simulink model "OL_HiLData"  (R2015b)
settings: Solver=FixedStepDiscrete  StartTime=0.0  StopTime=660  FixedStep=step_size  RelTol=1e-3
values from neighbouring files (symbols this model uses):
  step_size = 0.1    [loadCalib.m]
undefined symbols (not defined in the file or in its folder): canChannel, pack_current_eng, pack_current_raw, pack_voltage_eng, pack_voltage_raw, vehicle_voltage_eng, vehicle_voltage_raw
libraries: canmsglib x34, canlib x27, realtime_pacer_lib x1
(part 1 of 2)
settings Model: SimulationMode=accelerator  Creator=nctzv8  LastModifiedBy=nctzv8

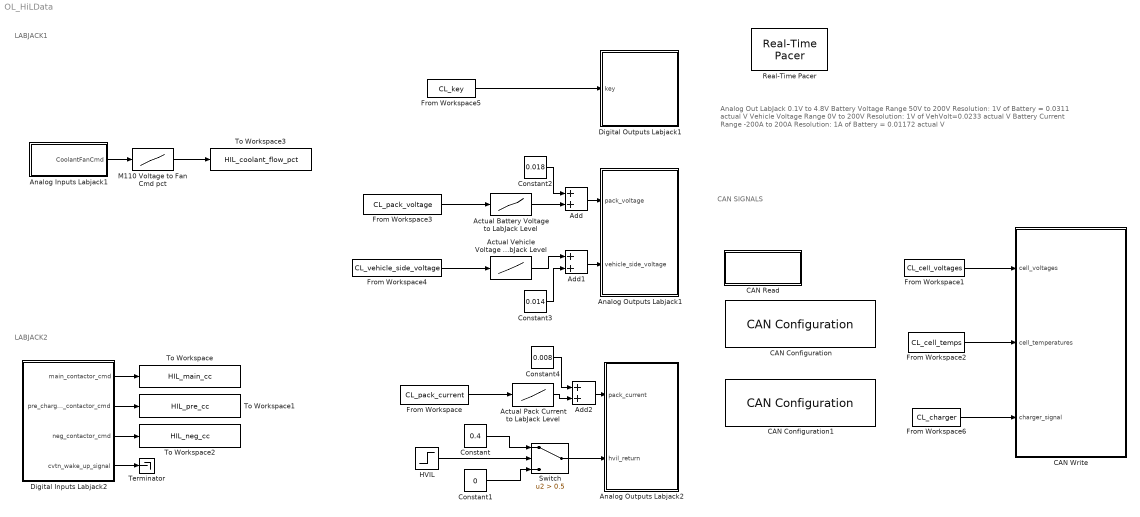
== system OL_HiLData ==
  note: CAN SIGNALS
  note: LABJACK2
  note: LABJACK1
  note: Analog Out LabJack 0.1V to 4.8V
      | Battery Voltage Range 50V to 200V Resolution: 1V of Battery = 0.0311 actual V
      | Vehicle Voltage Range 0V to 200V Resolution: 1V of VehVolt=0.0233 actual V
      | Battery Current Range -200A to 200A Resolution: 1A of Battery = 0.01172 actual V
  Actual Battery Voltage to LabJack Level : Lookup_n-D  NumberOfTableDimensions=1  BreakpointsForDimension1=pack_voltage_eng  Table=pack_voltage_raw  InternalRulePriority=Speed  RndMeth=Simplest  InputSameDT=on
  Actual Pack Current to LabJack Level : Lookup_n-D  NumberOfTableDimensions=1  BreakpointsForDimension1=pack_current_eng  Table=pack_current_raw  InternalRulePriority=Speed  RndMeth=Simplest  InputSameDT=on
  Actual Vehicle Voltage to LabJack Level : Lookup_n-D  NumberOfTableDimensions=1  BreakpointsForDimension1=vehicle_voltage_eng  Table=vehicle_voltage_raw  InternalRulePriority=Speed  RndMeth=Simplest  InputSameDT=on
  Add : Sum
  Add1 : Sum
  Add2 : Sum
  Analog Inputs Labjack1 : Subsystem
  Analog Outputs Labjack1 : Subsystem
  Analog Outputs Labjack2 : Subsystem
  CAN Configuration : canlib/CAN Configuration  BlockHandle=54.0011  DeviceMenu=Kvaser Virtual 1 (Channel 1)  Device=Kvaser USBcan Light 2 (Channel 1)  ObjConstructor=canChannel('Kvaser', 'USBcan Light 2', 1)  BusSpeed=500000  EnableBitParameters=off  SJW=1  TSEG1=4  TSEG2=3  NSamples=1  AckMode=Normal
  CAN Configuration1 : canlib/CAN Configuration  BlockHandle=55.0007  DeviceMenu=Kvaser Virtual 1 (Channel 1)  Device=Kvaser USBcan Light 2 (Channel 2)  ObjConstructor=canChannel('Kvaser', 'USBcan Light 2', 2)  BusSpeed=500000  EnableBitParameters=off  SJW=1  TSEG1=4  TSEG2=3  NSamples=1  AckMode=Normal
  CAN Read : Subsystem
  CAN Write : Subsystem
  Constant : Constant  Value=0.4  SampleTime=step_size
  Constant1 : Constant  Value=0  SampleTime=step_size
  Constant2 : Constant  Value=0.018  SampleTime=step_size
  Constant3 : Constant  Value=0.014  SampleTime=step_size
  Constant4 : Constant  Value=0.008  SampleTime=step_size
  Digital Inputs Labjack2 : Subsystem
  Digital Outputs Labjack1 : Subsystem
  From Workspace : FromWorkspace  VariableName=CL_pack_current  SampleTime=step_size
  From Workspace1 : FromWorkspace  VariableName=CL_cell_voltages  SampleTime=step_size
  From Workspace2 : FromWorkspace  VariableName=CL_cell_temps  SampleTime=step_size
  From Workspace3 : FromWorkspace  VariableName=CL_pack_voltage  SampleTime=step_size
  From Workspace4 : FromWorkspace  VariableName=CL_vehicle_side_voltage  SampleTime=step_size
  From Workspace5 : FromWorkspace  VariableName=CL_key  SampleTime=step_size
  From Workspace6 : FromWorkspace  VariableName=CL_charger  SampleTime=step_size
  HVIL : Step  Time=0  Before=1  SampleTime=step_size
  M110 Voltage to Fan Cmd pct : Lookup_n-D  NumberOfTableDimensions=1  BreakpointsForDimension1=[0 5]  Table=[0 100]  InternalRulePriority=Speed  RndMeth=Simplest  InputSameDT=on
  Real-Time Pacer : realtime_pacer_lib/Real-Time Pacer  simTimePerRealTime=1
  Switch : Switch  Criteria=u2 > Threshold  Threshold=0.5
  Terminator : Terminator
  To Workspace : ToWorkspace  VariableName=HIL_main_cc  SaveFormat=Timeseries  SampleTime=-1
  To Workspace1 : ToWorkspace  VariableName=HIL_pre_cc  SaveFormat=Timeseries  SampleTime=-1
  To Workspace2 : ToWorkspace  VariableName=HIL_neg_cc  SaveFormat=Timeseries  SampleTime=-1
  To Workspace3 : ToWorkspace  VariableName=HIL_coolant_flow_pct  SaveFormat=Timeseries  SampleTime=-1
  wires:
  From Workspace3/1 -> Actual Battery Voltage to LabJack Level/1
  From Workspace4/1 -> Actual Vehicle Voltage to LabJack Level/1
  From Workspace/1 -> Actual Pack Current to LabJack Level/1
  From Workspace5/1 -> Digital Outputs Labjack1/1(key)
  From Workspace1/1 -> CAN Write/1(cell_voltages)
  From Workspace2/1 -> CAN Write/2(cell_temperatures)
  HVIL/1 -> Switch/2
  Constant/1 -> Switch/1
  Constant1/1 -> Switch/3
  Switch/1 -> Analog Outputs Labjack2/2(hvil_return)
  Add/1 -> Analog Outputs Labjack1/1(pack_voltage)
  Actual Battery Voltage to LabJack Level/1 -> Add/2
  Constant2/1 -> Add/1
  Add1/1 -> Analog Outputs Labjack1/2(vehicle_side_voltage)
  Actual Vehicle Voltage to LabJack Level/1 -> Add1/1
  Constant3/1 -> Add1/2
  Add2/1 -> Analog Outputs Labjack2/1(pack_current)
  Actual Pack Current to LabJack Level/1 -> Add2/2
  Constant4/1 -> Add2/1
  Digital Inputs Labjack2/1(main_contactor_cmd) -> To Workspace/1
  Digital Inputs Labjack2/2(pre_charge_contactor_cmd) -> To Workspace1/1
  Digital Inputs Labjack2/3(neg_contactor_cmd) -> To Workspace2/1
  Digital Inputs Labjack2/4(cvtn_wake_up_signal) -> Terminator/1
  From Workspace6/1 -> CAN Write/3(charger_signal)
  Analog Inputs Labjack1/1(CoolantFanCmd) -> M110 Voltage to Fan Cmd pct/1
  M110 Voltage to Fan Cmd pct/1 -> To Workspace3/1

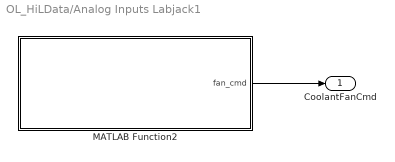
== system OL_HiLData/Analog Inputs Labjack1 ==
  MATLAB Function2 : MATLAB Function  TreatAsAtomicUnit=on
  CoolantFanCmd : Outport
  wires:
  MATLAB Function2/1(fan_cmd) -> CoolantFanCmd/1

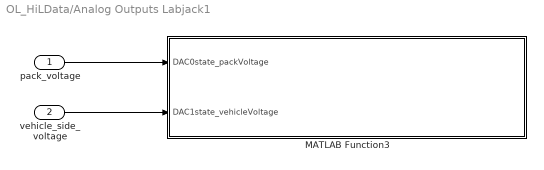
== system OL_HiLData/Analog Outputs Labjack1 ==
  pack_voltage : Inport
  vehicle_side_voltage : Inport  Port=2
  MATLAB Function3 : MATLAB Function  TreatAsAtomicUnit=on
  wires:
  pack_voltage/1 -> MATLAB Function3/1(DAC0state_packVoltage)
  vehicle_side_voltage/1 -> MATLAB Function3/2(DAC1state_vehicleVoltage)

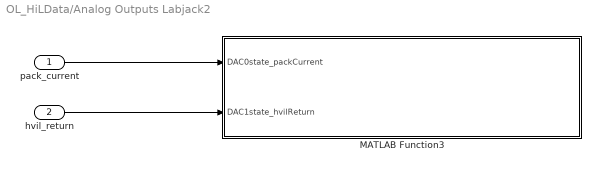
== system OL_HiLData/Analog Outputs Labjack2 ==
  pack_current : Inport
  hvil_return : Inport  Port=2
  MATLAB Function3 : MATLAB Function  TreatAsAtomicUnit=on
  wires:
  pack_current/1 -> MATLAB Function3/1(DAC0state_packCurrent)
  hvil_return/1 -> MATLAB Function3/2(DAC1state_hvilReturn)

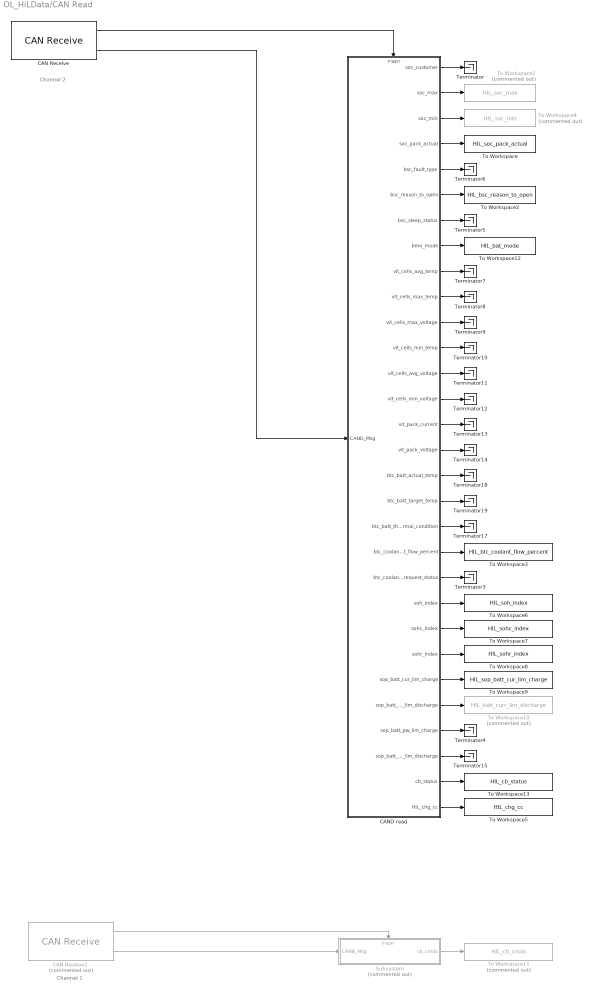
== system OL_HiLData/CAN Read ==
  note: Channel 1
  note: Channel 2
  CAN Receive : canlib/CAN Receive  BlockHandle=57.0007  DeviceMenu=Kvaser Virtual 1 (Channel 1)  Device=Kvaser USBcan Light 2 (Channel 2)  ObjConstructor=canChannel('Kvaser', 'USBcan Light 2', 2)  EnableStandardIDsFilter=off  StandardIDs=0  EnableExtendedIDsFilter=off  ExtendedIDs=0  SampleTime=step_size  MsgsPerTimestep=all  StdIDsCombo=Allow all  ExtIDsCombo=Allow all  InternalFilterUpdateStatus=on
  CAN Receive1 : canlib/CAN Receive  Commented=on  BlockHandle=58.0006  DeviceMenu=Kvaser Virtual 1 (Channel 1)  Device=Kvaser USBcan Light 2 (Channel 1)  ObjConstructor=canChannel('Kvaser', 'USBcan Light 2', 1)  EnableStandardIDsFilter=off  StandardIDs=0  EnableExtendedIDsFilter=off  ExtendedIDs=0  SampleTime=step_size  MsgsPerTimestep=all  StdIDsCombo=Allow all  ExtIDsCombo=Allow all  InternalFilterUpdateStatus=on
  CAND read : Subsystem
  Subsystem : Subsystem  Commented=on
  Terminator{,3..15,17..19} (17 alike) : Terminator
  To Workspace : ToWorkspace  VariableName=HIL_soc_pack_actual  SaveFormat=Timeseries  SampleTime=-1
  To Workspace1 : ToWorkspace  Commented=on  VariableName=HIL_soc_max  SaveFormat=Timeseries  SampleTime=-1
  To Workspace10 : ToWorkspace  Commented=on  VariableName=HIL_batt_curr_lim_discharge  SaveFormat=Timeseries  SampleTime=-1
  To Workspace11 : ToWorkspace  Commented=on  VariableName=HIL_cb_cmds  SaveFormat=Timeseries  SampleTime=-1
  To Workspace12 : ToWorkspace  VariableName=HIL_bat_mode  SaveFormat=Timeseries  SampleTime=-1
  To Workspace13 : ToWorkspace  VariableName=HIL_cb_status  SaveFormat=Timeseries  SampleTime=-1
  To Workspace2 : ToWorkspace  VariableName=HIL_bsc_reason_to_open  SaveFormat=Timeseries  SampleTime=-1
  To Workspace3 : ToWorkspace  VariableName=HIL_btc_coolant_flow_percent  SaveFormat=Timeseries  SampleTime=-1
  To Workspace4 : ToWorkspace  Commented=on  VariableName=HIL_soc_min  SaveFormat=Timeseries  SampleTime=-1
  To Workspace5 : ToWorkspace  VariableName=HIL_chg_cc  SaveFormat=Timeseries  SampleTime=-1
  To Workspace6 : ToWorkspace  VariableName=HIL_soh_index  SaveFormat=Timeseries  SampleTime=-1
  To Workspace7 : ToWorkspace  VariableName=HIL_sohc_index  SaveFormat=Timeseries  SampleTime=-1
  To Workspace8 : ToWorkspace  VariableName=HIL_sohr_index  SaveFormat=Timeseries  SampleTime=-1
  To Workspace9 : ToWorkspace  VariableName=HIL_sop_batt_cur_lim_charge  SaveFormat=Timeseries  SampleTime=-1
  wires:
  CAN Receive/2 -> CAND read/1(CAND_Msg)
  CAND read/1(soc_customer) -> Terminator/1
  CAND read/2(soc_max) -> To Workspace1/1
  CAND read/3(soc_min) -> To Workspace4/1
  CAND read/4(soc_pack_actual) -> To Workspace/1
  CAND read/5(bsc_fault_type) -> Terminator6/1
  CAND read/6(bsc_reason_to_open) -> To Workspace2/1
  CAND read/7(bsc_sleep_status) -> Terminator5/1
  CAND read/8(bmo_mode) -> To Workspace12/1
  CAND read/9(vit_cells_avg_temp) -> Terminator7/1
  CAND read/10(vit_cells_max_temp) -> Terminator8/1
  CAND read/11(vit_cells_max_voltage) -> Terminator9/1
  CAND read/12(vit_cells_min_temp) -> Terminator10/1
  CAND read/13(vit_cells_avg_voltage) -> Terminator11/1
  CAND read/14(vit_cells_min_voltage) -> Terminator12/1
  CAND read/15(vit_pack_current) -> Terminator13/1
  CAND read/16(vit_pack_voltage) -> Terminator14/1
  CAND read/17(btc_batt_actual_temp) -> Terminator18/1
  CAND read/18(btc_batt_target_temp) -> Terminator19/1
  CAND read/19(btc_batt_thermal_condition) -> Terminator17/1
  CAND read/20(btc_coolant_flow_percent) -> To Workspace3/1
  CAND read/21(btc_coolant_request_status) -> Terminator3/1
  CAND read/22(soh_index) -> To Workspace6/1
  CAND read/23(sohc_index) -> To Workspace7/1
  CAND read/24(sohr_index) -> To Workspace8/1
  CAND read/25(sop_batt_cur_lim_charge) -> To Workspace9/1
  CAND read/26(sop_batt_curr_lim_discharge) -> To Workspace10/1
  CAND read/27(sop_batt_pw_lim_charge) -> Terminator4/1
  CAND read/28(sop_batt_pw_lim_discharge) -> Terminator15/1
  CAND read/29(cb_status) -> To Workspace13/1
  CAN Receive1/1 -> Subsystem/Trigger
  CAN Receive1/2 -> Subsystem/1(CANB_Msg)
  Subsystem/1(cb_cmds) -> To Workspace11/1
  CAND read/30(HIL_chg_cc) -> To Workspace5/1
  CAN Receive/1 -> CAND read/Trigger

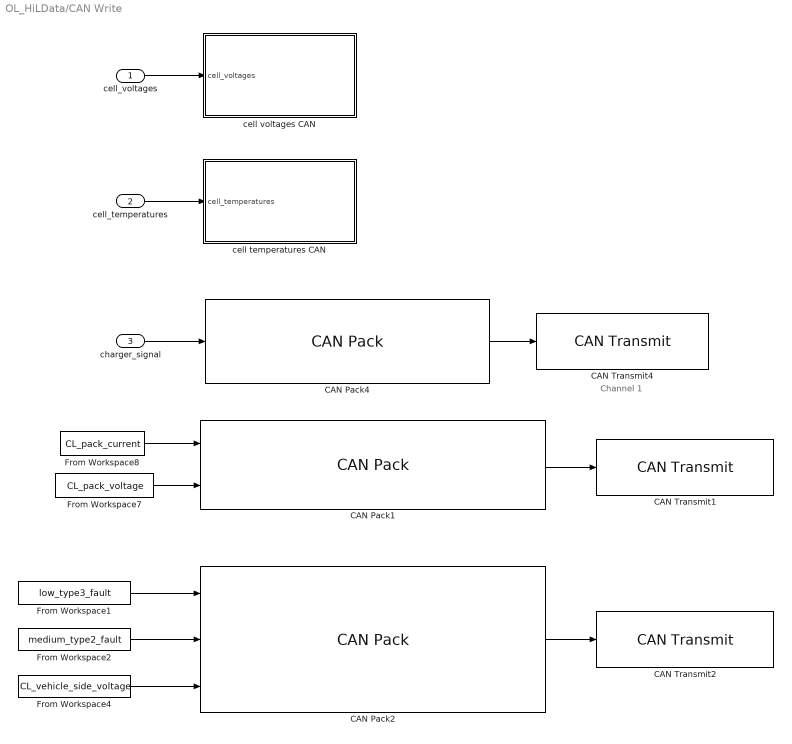
== system OL_HiLData/CAN Write ==
  note: Channel 1
  cell_voltages : Inport
  cell_temperatures : Inport  Port=2
  charger_signal : Inport  Port=3
  CAN Pack1 : canmsglib/CAN Pack  CANdbFile=C:\Sagar\Projects\BMS\P006n\08_Work_in_progress\WP3_2_BMS_Stage_1\OpenLoopDataSend\BMSdb.dbc  MsgList=pack_data  MsgName=pack_data  MsgIDType=Standard (11-bit identifier)  MsgIdentifier=36  MsgLength=8  SignalInfo=pack_current$16$24$2$1$1$0$1.000000e-03$0$-200$200$#pack_voltage$40$24$2$2$1$0$1.000000e-03$0$0$200$#  NSignals=2  StartBits=str2num('[int32(16);int32(40)]')  SignalSizes=str2num('[int32(24);int32(24)]')  ByteOrders=str2num('[int32(2);int32(2)]')  DataTypes=str2num('[int32(1);int32(2)]')  MultiplexTypes=str2num('[int32(1);int32(1)]')  MultiplexValues=str2num('[double(0);double(0)]')  Factors=str2num('[double(1.000000e-03);double(1.000000e-03)]')  Offsets=str2num('[double(0);double(0)]')  Minimums=str2num('[double(-200);double(0)]')  Maximums=str2num('[double(200);double(200)]')  Remote=off
      settings: DataFormat=CANdb specified signals
  CAN Pack2 : canmsglib/CAN Pack  CANdbFile=C:\Sagar\Projects\BMS\P006n\08_Work_in_progress\WP3_2_BMS_Stage_1\OpenLoopDataSend\BMSdb.dbc  MsgList=pack_data_2  MsgName=pack_data_2  MsgIDType=Standard (11-bit identifier)  MsgIdentifier=37  MsgLength=8  SignalInfo=low_fault$30$1$2$2$1$0$1$0$0$1$#medium_fault$31$1$2$2$1$0$1$0$0$1$#vehicle_side_voltage$16$24$2$2$1$0$1$0$0$200$#  NSignals=3  StartBits=str2num('[int32(30);int32(31);int32(16)]')  SignalSizes=str2num('[int32(1);int32(1);int32(24)]')  ByteOrders=str2num('[int32(2);int32(2);int32(2)]')  DataTypes=str2num('[int32(2);int32(2);int32(2)]')  MultiplexTypes=str2num('[int32(1);int32(1);int32(1)]')  MultiplexValues=str2num('[double(0);double(0);double(0)]')  Factors=str2num('[double(1);double(1);double(1)]')  Offsets=str2num('[double(0);double(0);double(0)]')  Minimums=str2num('[double(0);double(0);double(0)]')  Maximums=str2num('[double(1);double(1);double(200)]')  Remote=off
      settings: DataFormat=CANdb specified signals
  CAN Pack4 : canmsglib/CAN Pack  CANdbFile=C:\Sagar\Projects\BMS\P006n\08_Work_in_progress\WP3_2_BMS_Stage_1\OpenLoopDataSend\BMSdb.dbc  MsgList=socket_charging  MsgName=socket_charging  MsgIDType=Standard (11-bit identifier)  MsgIdentifier=35  MsgLength=8  SignalInfo=charger_signal$7$1$2$2$1$0$1$0$0$1$#  NSignals=1  StartBits=str2num('[int32(7)]')  SignalSizes=str2num('[int32(1)]')  ByteOrders=str2num('[int32(2)]')  DataTypes=str2num('[int32(2)]')  MultiplexTypes=str2num('[int32(1)]')  MultiplexValues=str2num('[double(0)]')  Factors=str2num('[double(1)]')  Offsets=str2num('[double(0)]')  Minimums=str2num('[double(0)]')  Maximums=str2num('[double(1)]')  Remote=off
      settings: DataFormat=CANdb specified signals
  CAN Transmit1 : canlib/CAN Transmit  BlockHandle=300.0009  DeviceMenu=Kvaser Virtual 1 (Channel 1)  Device=Kvaser USBcan Light 2 (Channel 1)  ObjConstructor=canChannel('Kvaser', 'USBcan Light 2', 1)  EnablePeriodicTransmit=off  MessagePeriod=1.000
  CAN Transmit2 : canlib/CAN Transmit  BlockHandle=301.0009  DeviceMenu=Kvaser Virtual 1 (Channel 1)  Device=Kvaser USBcan Light 2 (Channel 1)  ObjConstructor=canChannel('Kvaser', 'USBcan Light 2', 1)  EnablePeriodicTransmit=off  MessagePeriod=1.000
  CAN Transmit4 : canlib/CAN Transmit  BlockHandle=302.0009  DeviceMenu=Kvaser Virtual 1 (Channel 1)  Device=Kvaser USBcan Light 2 (Channel 1)  ObjConstructor=canChannel('Kvaser', 'USBcan Light 2', 1)  EnablePeriodicTransmit=off  MessagePeriod=1.000
  From Workspace1 : FromWorkspace  VariableName=low_type3_fault  SampleTime=step_size
  From Workspace2 : FromWorkspace  VariableName=medium_type2_fault  SampleTime=step_size
  From Workspace4 : FromWorkspace  VariableName=CL_vehicle_side_voltage  SampleTime=step_size
  From Workspace7 : FromWorkspace  VariableName=CL_pack_voltage  SampleTime=step_size
  From Workspace8 : FromWorkspace  VariableName=CL_pack_current  SampleTime=step_size
  cell temperatures CAN : Subsystem
  cell voltages CAN : Subsystem
  wires:
  cell_voltages/1 -> cell voltages CAN/1(cell_voltages)
  cell_temperatures/1 -> cell temperatures CAN/1(cell_temperatures)
  CAN Pack4/1 -> CAN Transmit4/1
  charger_signal/1 -> CAN Pack4/1
  CAN Pack1/1 -> CAN Transmit1/1
  From Workspace8/1 -> CAN Pack1/1
  From Workspace7/1 -> CAN Pack1/2
  CAN Pack2/1 -> CAN Transmit2/1
  From Workspace4/1 -> CAN Pack2/3
  From Workspace1/1 -> CAN Pack2/1
  From Workspace2/1 -> CAN Pack2/2

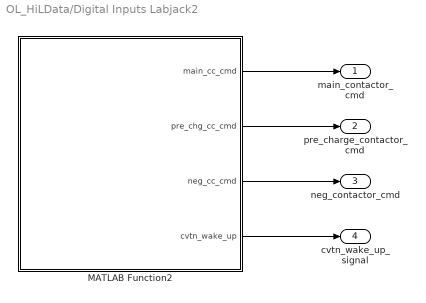
== system OL_HiLData/Digital Inputs Labjack2 ==
  MATLAB Function2 : MATLAB Function  TreatAsAtomicUnit=on
  main_contactor_cmd : Outport
  pre_charge_contactor_cmd : Outport  Port=2
  neg_contactor_cmd : Outport  Port=3
  cvtn_wake_up_signal : Outport  Port=4
  wires:
  MATLAB Function2/1(main_cc_cmd) -> main_contactor_cmd/1
  MATLAB Function2/2(pre_chg_cc_cmd) -> pre_charge_contactor_cmd/1
  MATLAB Function2/3(neg_cc_cmd) -> neg_contactor_cmd/1
  MATLAB Function2/4(cvtn_wake_up) -> cvtn_wake_up_signal/1

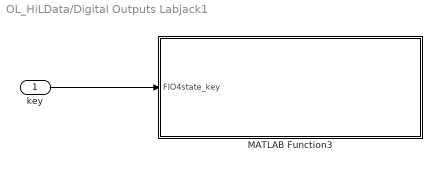
== system OL_HiLData/Digital Outputs Labjack1 ==
  key : Inport
  MATLAB Function3 : MATLAB Function  TreatAsAtomicUnit=on
  wires:
  key/1 -> MATLAB Function3/1(FIO4state_key)

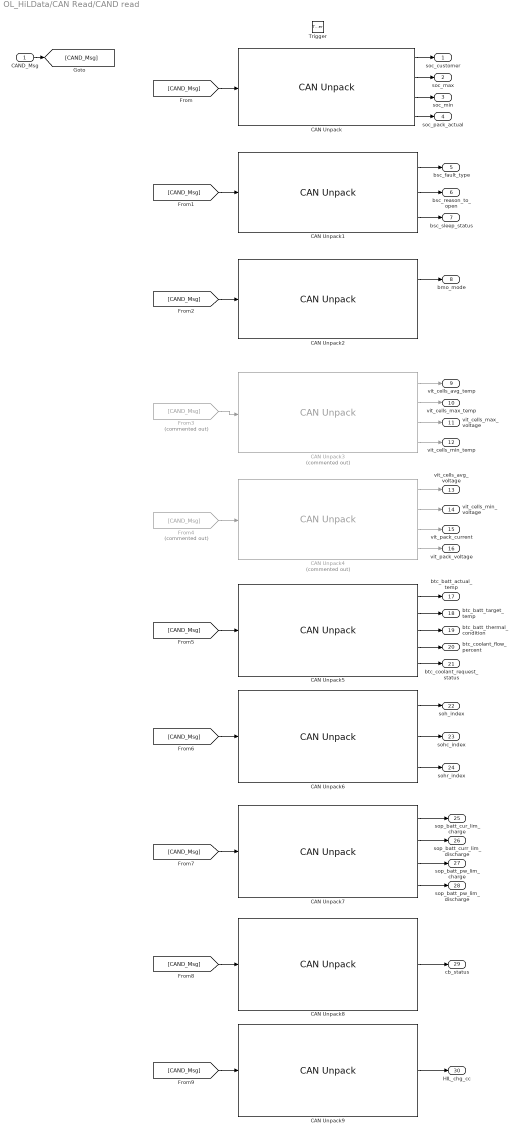
== system OL_HiLData/CAN Read/CAND read ==
  CAND_Msg : Inport
  Trigger : TriggerPort  TriggerType=function-call  PortDimensions=1
  CAN Unpack : canmsglib/CAN Unpack  CANdbFile=C:\Sagar\Projects\BMS\P006n\08_Work_in_progress\WP3_2_BMS_Stage_1\OpenLoopDataSend\VEHdb.dbc  MsgList=soc_info  MsgName=soc_info  MsgIDType=Standard (11-bit identifier)  MsgIdentifier=2  MsgLength=8  SignalInfo=soc_customer$8$16$2$2$1$0$1.000000e-02$0$0$100$#soc_max$56$16$2$2$1$0$1.000000e-02$0$0$100$#soc_min$40$16$2$2$1$0$1.000000e-02$0$0$100$#soc_pack_actual$24$16$2$2$1$0$1.000000e-02$0$0$100$#  NSignals=4  IDPort=off  TimestampPort=off  ErrorPort=off  RemotePort=off  LengthPort=off  StatusPort=off  StartBits=str2num('[int32(8);int32(56);int32(40);int32(24)]')  SignalSizes=str2num('[int32(16);int32(16);int32(16);int32(16)]')  ByteOrders=str2num('[int32(2);int32(2);int32(2);int32(2)]')  DataTypes=str2num('[int32(2);int32(2);int32(2);int32(2)]')  MultiplexTypes=str2num('[int32(1);int32(1);int32(1);int32(1)]')  MultiplexValues=str2num('[double(0);double(0);double(0);double(0)]')  Factors=str2num('[double(1.000000e-02);double(1.000000e-02);double(1.000000e-02);double(1.000000e-02)]')  Offsets=str2num('[double(0);double(0);double(0);double(0)]')  Minimums=str2num('[double(0);double(0);double(0);double(0)]')  Maximums=str2num('[double(100);double(100);double(100);double(100)]')
      settings: DataFormat=CANdb specified signals
  CAN Unpack1 : canmsglib/CAN Unpack  CANdbFile=C:\Sagar\Projects\BMS\P006n\08_Work_in_progress\WP3_2_BMS_Stage_1\OpenLoopDataSend\VEHdb.dbc  MsgList=bsc_info  MsgName=bsc_info  MsgIDType=Standard (11-bit identifier)  MsgIdentifier=3  MsgLength=8  SignalInfo=bsc_fault_type$8$8$2$2$1$0$1$0$0$20$#bsc_reason_to_open$0$8$2$2$1$0$1$0$0$20$#bsc_sleep_status$23$1$2$2$1$0$1$0$0$1$#  NSignals=3  IDPort=off  TimestampPort=off  ErrorPort=off  RemotePort=off  LengthPort=off  StatusPort=off  StartBits=str2num('[int32(8);int32(0);int32(23)]')  SignalSizes=str2num('[int32(8);int32(8);int32(1)]')  ByteOrders=str2num('[int32(2);int32(2);int32(2)]')  DataTypes=str2num('[int32(2);int32(2);int32(2)]')  MultiplexTypes=str2num('[int32(1);int32(1);int32(1)]')  MultiplexValues=str2num('[double(0);double(0);double(0)]')  Factors=str2num('[double(1);double(1);double(1)]')  Offsets=str2num('[double(0);double(0);double(0)]')  Minimums=str2num('[double(0);double(0);double(0)]')  Maximums=str2num('[double(20);double(20);double(1)]')
      settings: DataFormat=CANdb specified signals
  CAN Unpack2 : canmsglib/CAN Unpack  CANdbFile=C:\Sagar\Projects\BMS\P006n\08_Work_in_progress\WP3_2_BMS_Stage_1\OpenLoopDataSend\VEHdb.dbc  MsgList=bmo_info  MsgName=bmo_info  MsgIDType=Standard (11-bit identifier)  MsgIdentifier=4  MsgLength=8  SignalInfo=bmo_mode$0$8$2$2$1$0$1$0$0$10$#soc_rate_high$15$1$2$2$1$0$1$0$0$1$#  NSignals=2  IDPort=off  TimestampPort=off  ErrorPort=off  RemotePort=off  LengthPort=off  StatusPort=off  StartBits=str2num('[int32(0);int32(15)]')  SignalSizes=str2num('[int32(8);int32(1)]')  ByteOrders=str2num('[int32(2);int32(2)]')  DataTypes=str2num('[int32(2);int32(2)]')  MultiplexTypes=str2num('[int32(1);int32(1)]')  MultiplexValues=str2num('[double(0);double(0)]')  Factors=str2num('[double(1);double(1)]')  Offsets=str2num('[double(0);double(0)]')  Minimums=str2num('[double(0);double(0)]')  Maximums=str2num('[double(10);double(1)]')
      settings: DataFormat=CANdb specified signals
  CAN Unpack3 : canmsglib/CAN Unpack  Commented=on  CANdbFile=C:\Sagar\Projects\BMS\P006n\08_Work_in_progress\WP3_2_BMS_Stage_1\OpenLoopDataSend\VEHdb.dbc  MsgList=vit_info1  MsgName=vit_info1  MsgIDType=Standard (11-bit identifier)  MsgIdentifier=5  MsgLength=8  SignalInfo=vit_cells_avg_temp$40$16$2$1$1$0$1.000000e-02$0$-100$120$#vit_cells_max_temp$8$16$2$1$1$0$1.000000e-02$0$-100$120$#vit_cells_max_voltage$56$16$2$2$1$0$1.000000e-02$0$0$5$#vit_cells_min_temp$24$16$2$1$1$0$1.000000e-02$0$-100$120$#  NSignals=4  IDPort=off  TimestampPort=off  ErrorPort=off  RemotePort=off  LengthPort=off  StatusPort=off  StartBits=str2num('[int32(40);int32(8);int32(56);int32(24)]')  SignalSizes=str2num('[int32(16);int32(16);int32(16);int32(16)]')  ByteOrders=str2num('[int32(2);int32(2);int32(2);int32(2)]')  DataTypes=str2num('[int32(1);int32(1);int32(2);int32(1)]')  MultiplexTypes=str2num('[int32(1);int32(1);int32(1);int32(1)]')  MultiplexValues=str2num('[double(0);double(0);double(0);double(0)]')  Factors=str2num('[double(1.000000e-02);double(1.000000e-02);double(1.000000e-02);double(1.000000e-02)]')  Offsets=str2num('[double(0);double(0);double(0);double(0)]')  Minimums=str2num('[double(-100);double(-100);double(0);double(-100)]')  Maximums=str2num('[double(120);double(120);double(5);double(120)]')
      settings: DataFormat=CANdb specified signals
  CAN Unpack4 : canmsglib/CAN Unpack  Commented=on  CANdbFile=C:\Sagar\Projects\BMS\P006n\08_Work_in_progress\WP3_2_BMS_Stage_1\OpenLoopDataSend\VEHdb.dbc  MsgList=vit_info2  MsgName=vit_info2  MsgIDType=Standard (11-bit identifier)  MsgIdentifier=6  MsgLength=8  SignalInfo=vit_cells_avg_voltage$24$16$2$2$1$0$1.000000e-02$0$0$5$#vit_cells_min_voltage$8$16$2$2$1$0$1.000000e-02$0$0$5$#vit_pack_current$56$16$2$1$1$0$1.000000e-02$0$-300$300$#vit_pack_voltage$40$16$2$2$1$0$1.000000e-02$0$0$200$#  NSignals=4  IDPort=off  TimestampPort=off  ErrorPort=off  RemotePort=off  LengthPort=off  StatusPort=off  StartBits=str2num('[int32(24);int32(8);int32(56);int32(40)]')  SignalSizes=str2num('[int32(16);int32(16);int32(16);int32(16)]')  ByteOrders=str2num('[int32(2);int32(2);int32(2);int32(2)]')  DataTypes=str2num('[int32(2);int32(2);int32(1);int32(2)]')  MultiplexTypes=str2num('[int32(1);int32(1);int32(1);int32(1)]')  MultiplexValues=str2num('[double(0);double(0);double(0);double(0)]')  Factors=str2num('[double(1.000000e-02);double(1.000000e-02);double(1.000000e-02);double(1.000000e-02)]')  Offsets=str2num('[double(0);double(0);double(0);double(0)]')  Minimums=str2num('[double(0);double(0);double(-300);double(0)]')  Maximums=str2num('[double(5);double(5);double(300);double(200)]')
      settings: DataFormat=CANdb specified signals
  CAN Unpack5 : canmsglib/CAN Unpack  CANdbFile=C:\Sagar\Projects\BMS\P006n\08_Work_in_progress\WP3_2_BMS_Stage_1\OpenLoopDataSend\VEHdb.dbc  MsgList=btc_info  MsgName=btc_info  MsgIDType=Standard (11-bit identifier)  MsgIdentifier=7  MsgLength=8  SignalInfo=btc_batt_actual_temp$16$16$2$1$1$0$5.000000e-01$0$-50$80$#btc_batt_target_temp$40$16$2$1$1$0$5.000000e-01$0$-50$80$#btc_batt_thermal_condition$6$1$2$2$1$0$1$0$0$1$#btc_coolant_flow_percent$24$8$2$2$1$0$1$0$0$100$#btc_coolant_request_status$7$1$2$2$1$0$1$0$0$1$#  NSignals=5  IDPort=off  TimestampPort=off  ErrorPort=off  RemotePort=off  LengthPort=off  StatusPort=off  StartBits=str2num('[int32(16);int32(40);int32(6);int32(24);int32(7)]')  SignalSizes=str2num('[int32(16);int32(16);int32(1);int32(8);int32(1)]')  ByteOrders=str2num('[int32(2);int32(2);int32(2);int32(2);int32(2)]')  DataTypes=str2num('[int32(1);int32(1);int32(2);int32(2);int32(2)]')  MultiplexTypes=str2num('[int32(1);int32(1);int32(1);int32(1);int32(1)]')  MultiplexValues=str2num('[double(0);double(0);double(0);double(0);double(0)]')  Factors=str2num('[double(5.000000e-01);double(5.000000e-01);double(1);double(1);double(1)]')  Offsets=str2num('[double(0);double(0);double(0);double(0);double(0)]')  Minimums=str2num('[double(-50);double(-50);double(0);double(0);double(0)]')  Maximums=str2num('[double(80);double(80);double(1);double(100);double(1)]')
      settings: DataFormat=CANdb specified signals
  CAN Unpack6 : canmsglib/CAN Unpack  CANdbFile=C:\Sagar\Projects\BMS\P006n\08_Work_in_progress\WP3_2_BMS_Stage_1\OpenLoopDataSend\VEHdb.dbc  MsgList=soh_info  MsgName=soh_info  MsgIDType=Standard (11-bit identifier)  MsgIdentifier=8  MsgLength=8  SignalInfo=soh_index$8$16$2$2$1$0$1.000000e-02$0$0$100$#sohc_index$40$16$2$2$1$0$1.000000e-02$0$0$100$#sohr_index$24$16$2$2$1$0$1.000000e-02$0$0$100$#  NSignals=3  IDPort=off  TimestampPort=off  ErrorPort=off  RemotePort=off  LengthPort=off  StatusPort=off  StartBits=str2num('[int32(8);int32(40);int32(24)]')  SignalSizes=str2num('[int32(16);int32(16);int32(16)]')  ByteOrders=str2num('[int32(2);int32(2);int32(2)]')  DataTypes=str2num('[int32(2);int32(2);int32(2)]')  MultiplexTypes=str2num('[int32(1);int32(1);int32(1)]')  MultiplexValues=str2num('[double(0);double(0);double(0)]')  Factors=str2num('[double(1.000000e-02);double(1.000000e-02);double(1.000000e-02)]')  Offsets=str2num('[double(0);double(0);double(0)]')  Minimums=str2num('[double(0);double(0);double(0)]')  Maximums=str2num('[double(100);double(100);double(100)]')
      settings: DataFormat=CANdb specified signals
  CAN Unpack7 : canmsglib/CAN Unpack  CANdbFile=C:\Sagar\Projects\BMS\P006n\08_Work_in_progress\WP3_2_BMS_Stage_1\OpenLoopDataSend\VEHdb.dbc  MsgList=sop_info  MsgName=sop_info  MsgIDType=Standard (11-bit identifier)  MsgIdentifier=9  MsgLength=8  SignalInfo=sop_batt_curr_lim_charge$40$16$2$2$1$0$5.000000e-02$0$0$512$#sop_batt_curr_lim_discharge$56$16$2$2$1$0$5.000000e-02$0$0$512$#sop_batt_pw_lim_charge$8$16$2$2$1$0$4$0$0$256000$#sop_batt_pw_lim_discharge$24$16$2$2$1$0$4$0$0$256000$#  NSignals=4  IDPort=off  TimestampPort=off  ErrorPort=off  RemotePort=off  LengthPort=off  StatusPort=off  StartBits=str2num('[int32(40);int32(56);int32(8);int32(24)]')  SignalSizes=str2num('[int32(16);int32(16);int32(16);int32(16)]')  ByteOrders=str2num('[int32(2);int32(2);int32(2);int32(2)]')  DataTypes=str2num('[int32(2);int32(2);int32(2);int32(2)]')  MultiplexTypes=str2num('[int32(1);int32(1);int32(1);int32(1)]')  MultiplexValues=str2num('[double(0);double(0);double(0);double(0)]')  Factors=str2num('[double(5.000000e-02);double(5.000000e-02);double(4);double(4)]')  Offsets=str2num('[double(0);double(0);double(0);double(0)]')  Minimums=str2num('[double(0);double(0);double(0);double(0)]')  Maximums=str2num('[double(512);double(512);double(256000);double(256000)]')
      settings: DataFormat=CANdb specified signals
  CAN Unpack8 : canmsglib/CAN Unpack  CANdbFile=C:\Sagar\Projects\BMS\P006n\08_Work_in_progress\WP3_2_BMS_Stage_1\OpenLoopDataSend\VEHdb.dbc  MsgList=cb_info  MsgName=cb_info  MsgIDType=Standard (11-bit identifier)  MsgIdentifier=16  MsgLength=8  SignalInfo=cb_status$7$1$2$2$1$0$1$0$0$1$#  NSignals=1  IDPort=off  TimestampPort=off  ErrorPort=off  RemotePort=off  LengthPort=off  StatusPort=off  StartBits=str2num('[int32(7)]')  SignalSizes=str2num('[int32(1)]')  ByteOrders=str2num('[int32(2)]')  DataTypes=str2num('[int32(2)]')  MultiplexTypes=str2num('[int32(1)]')  MultiplexValues=str2num('[double(0)]')  Factors=str2num('[double(1)]')  Offsets=str2num('[double(0)]')  Minimums=str2num('[double(0)]')  Maximums=str2num('[double(1)]')
      settings: DataFormat=CANdb specified signals
  CAN Unpack9 : canmsglib/CAN Unpack  CANdbFile=C:\Sagar\Projects\BMS\P006n\08_Work_in_progress\WP3_2_BMS_Stage_1\OpenLoopDataSend\VEHdb.dbc  MsgList=socket_charging_contactor  MsgName=socket_charging_contactor  MsgIDType=Standard (11-bit identifier)  MsgIdentifier=17  MsgLength=8  SignalInfo=charger_contactor$7$1$2$2$1$0$1$0$0$1$#  NSignals=1  IDPort=off  TimestampPort=off  ErrorPort=off  RemotePort=off  LengthPort=off  StatusPort=off  StartBits=str2num('[int32(7)]')  SignalSizes=str2num('[int32(1)]')  ByteOrders=str2num('[int32(2)]')  DataTypes=str2num('[int32(2)]')  MultiplexTypes=str2num('[int32(1)]')  MultiplexValues=str2num('[double(0)]')  Factors=str2num('[double(1)]')  Offsets=str2num('[double(0)]')  Minimums=str2num('[double(0)]')  Maximums=str2num('[double(1)]')
      settings: DataFormat=CANdb specified signals
  From3 : From  Commented=on  GotoTag=CAND_Msg
  From4 : From  Commented=on  GotoTag=CAND_Msg
  soc_customer : Outport
  soc_max : Outport  Port=2
  soc_min : Outport  Port=3
  soc_pack_actual : Outport  Port=4
  bsc_fault_type : Outport  Port=5
  bsc_reason_to_open : Outport  Port=6
  bsc_sleep_status : Outport  Port=7
  bmo_mode : Outport  Port=8
  vit_cells_avg_temp : Outport  Port=9
  vit_cells_max_temp : Outport  Port=10
  vit_cells_max_voltage : Outport  Port=11
  vit_cells_min_temp : Outport  Port=12
  vit_cells_avg_voltage : Outport  Port=13
  vit_cells_min_voltage : Outport  Port=14
  vit_pack_current : Outport  Port=15
  vit_pack_voltage : Outport  Port=16
  btc_batt_actual_temp : Outport  Port=17
  btc_batt_target_temp : Outport  Port=18
  btc_batt_thermal_condition : Outport  Port=19
  btc_coolant_flow_percent : Outport  Port=20
  btc_coolant_request_status : Outport  Port=21
  soh_index : Outport  Port=22
  sohc_index : Outport  Port=23
  sohr_index : Outport  Port=24
  sop_batt_cur_lim_charge : Outport  Port=25
  sop_batt_curr_lim_discharge : Outport  Port=26
  sop_batt_pw_lim_charge : Outport  Port=27
  sop_batt_pw_lim_discharge : Outport  Port=28
  cb_status : Outport  Port=29
  HIL_chg_cc : Outport  Port=30
  wires:
  CAN Unpack/1 -> soc_customer/1
  CAN Unpack/2 -> soc_max/1
  CAN Unpack/3 -> soc_min/1
  CAN Unpack/4 -> soc_pack_actual/1
  CAND_Msg/1 -> [CAND_Msg]
  [CAND_Msg] -> CAN Unpack/1
  [CAND_Msg] -> CAN Unpack1/1
  CAN Unpack1/1 -> bsc_fault_type/1
  CAN Unpack1/2 -> bsc_reason_to_open/1
  CAN Unpack1/3 -> bsc_sleep_status/1
  [CAND_Msg] -> CAN Unpack2/1
  CAN Unpack2/1 -> bmo_mode/1
  From3/1 -> CAN Unpack3/1
  CAN Unpack3/1 -> vit_cells_avg_temp/1
  CAN Unpack3/2 -> vit_cells_max_temp/1
  CAN Unpack3/3 -> vit_cells_max_voltage/1
  CAN Unpack3/4 -> vit_cells_min_temp/1
  From4/1 -> CAN Unpack4/1
  CAN Unpack4/1 -> vit_cells_avg_voltage/1
  CAN Unpack4/2 -> vit_cells_min_voltage/1
  CAN Unpack4/3 -> vit_pack_current/1
  CAN Unpack4/4 -> vit_pack_voltage/1
  [CAND_Msg] -> CAN Unpack5/1
  CAN Unpack5/1 -> btc_batt_actual_temp/1
  CAN Unpack5/2 -> btc_batt_target_temp/1
  CAN Unpack5/3 -> btc_batt_thermal_condition/1
  CAN Unpack5/4 -> btc_coolant_flow_percent/1
  CAN Unpack5/5 -> btc_coolant_request_status/1
  [CAND_Msg] -> CAN Unpack6/1
  CAN Unpack6/1 -> soh_index/1
  [CAND_Msg] -> CAN Unpack7/1
  CAN Unpack7/1 -> sop_batt_cur_lim_charge/1
  CAN Unpack7/2 -> sop_batt_curr_lim_discharge/1
  CAN Unpack7/3 -> sop_batt_pw_lim_charge/1
  CAN Unpack7/4 -> sop_batt_pw_lim_discharge/1
  [CAND_Msg] -> CAN Unpack8/1
  CAN Unpack8/1 -> cb_status/1
  CAN Unpack6/3 -> sohr_index/1
  CAN Unpack6/2 -> sohc_index/1
  [CAND_Msg] -> CAN Unpack9/1
  CAN Unpack9/1 -> HIL_chg_cc/1

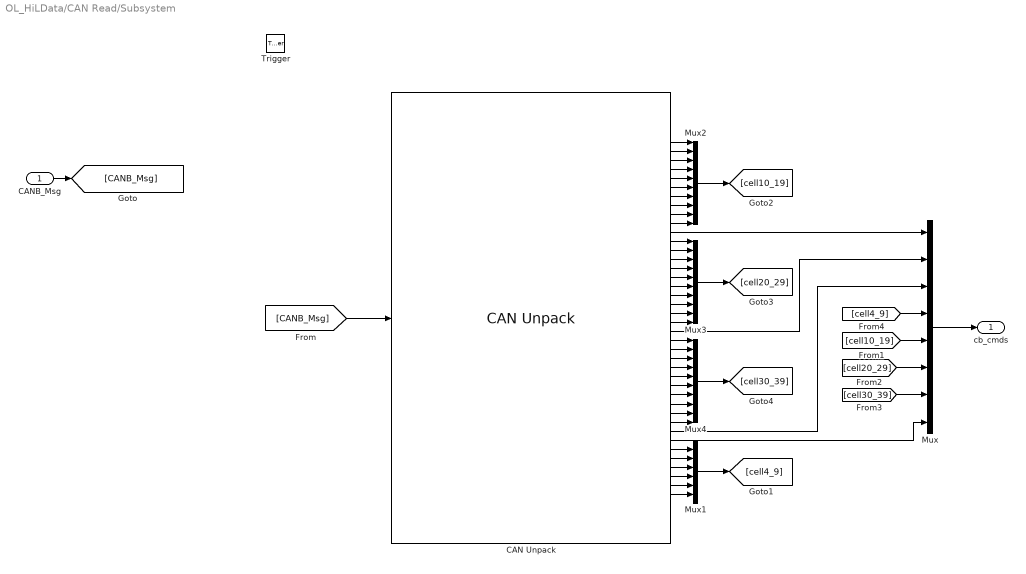
== system OL_HiLData/CAN Read/Subsystem ==
  CANB_Msg : Inport
  Trigger : TriggerPort  TriggerType=function-call  PortDimensions=1
  CAN Unpack : canmsglib/CAN Unpack  CANdbFile=C:\Sagar\Projects\BMS\P006n\08_Work_in_progress\WP3_2_BMS_Stage_1\OpenLoopDataSend\BMSdb.dbc  MsgList=cell_bal_cmd  MsgName=cell_bal_cmd  MsgIDType=Standard (11-bit identifier)  MsgIdentifier=23  MsgLength=8  SignalInfo=cell10_cb_cmd$14$1$2$2$1$0$1$0$0$1$#cell11_cb_cmd$13$1$2$2$1$0$1$0$0$1$#cell12_cb_cmd$12$1$2$2$1$0$1$0$0$1$#cell13_cb_cmd$11$1$2$2$1$0$1$0$0$1$#cell14_cb_cmd$10$1$2$2$1$0$1$0$0$1$#cell15_cb_cmd$9$1$2$2$1$0$1$0$0$1$#cell16_cb_cmd$8$1$2$2$1$0$1$0$0$1$#cell17_cb_cmd$23$1$2$2$1$0$1$0$0$1$#cell18_cb_cmd$22$1$2$2$1$0$1$0$0$1$#cell19_cb_cmd$21$1$2$2$1$0$1$0$0$1$#cell1_cb_cmd$7$1$2$2$1$0$1$0$0$1$#cell20_cb_cmd$20$1$2$2$1$0$1$0$0$1$#cell21_cb_cmd$19$1$2$2$1$0$1$0$0$1$#cell22_cb_cmd$18$1$2$2$1$0$1$0$0$1$#cell23_cb_cmd$17$1$2$2$1$0$1$0$0$1$#cell24_cb_cmd$16$1$2$2$1$0$1$0$0$1$#cell25_cb_cmd$31$1$2$2$1$0$1$0$0$1$#cell26_cb_cmd$30$1$2$2$1$0$1$0$0$1$#cell27_cb_cmd$29$1$2$2$1$0$1$0$0$1$#cell28_cb_cmd$28$1$2$2$1$0$1$0$0$1$#cell29_cb_cmd$27$1$2$2$1$0$1$0$0$1$#cell2_cb_cmd$6$1$2$2$1$0$1$0$0$1$#cell30_cb_cmd$26$1$2$2$1$0$1$0$0$1$#cell31_cb_cmd$25$1$2$2$1$0$1$0$0$1$#cell32_cb_cmd$24$1$2$2$1$0$1$0$0$1$#cell33_cb_cmd$39$1$2$2$1$0$1$0$0$1$#cell34_cb_cmd$38$1$2$2$1$0$1$0$0$1$#cell35_cb_cmd$37$1$2$2$1$0$1$0$0$1$#cell36_cb_cmd$36$1$2$2$1$0$1$0$0$1$#cell37_cb_cmd$35$1$2$2$1$0$1$0$0$1$#cell38_cb_cmd$34$1$2$2$1$0$1$0$0$1$#cell39_cb_cmd$33$1$2$2$1$0$1$0$0$1$#cell3_cb_cmd$5$1$2$2$1$0$1$0$0$1$#cell40_cb_cmd$32$1$2$2$1$0$1$0$0$1$#cell4_cb_cmd$4$1$2$2$1$0$1$0$0$1$#cell5_cb_cmd$3$1$2$2$1$0$1$0$0$1$#cell6_cb_cmd$2$1$2$2$1$0$1$0$0$1$#cell7_cb_cmd$1$1$2$2$1$0$1$0$0$1$#cell8_cb_cmd$0$1$2$2$1$0$1$0$0$1$#cell9_cb_cmd$15$1$2$2$1$0$1$0$0$1$#  NSignals=40  IDPort=off  TimestampPort=off  ErrorPort=off  RemotePort=off  LengthPort=off  StatusPort=off  StartBits=str2num('[int32(14);int32(13);int32(12);int32(11);int32(10);int32(9);int32(8);int32(23);int32(22);int32(21);int32(7);int32(20);int32(19);int32(18);int32(17);int32(16);int32(31);int32(30);int32(29);int32(28);int32(27);int32(6);int32(26);int32(25);int32(24);int32(39);int32(38);int32(37);int32(36);int32(35);int32(34);int32(33);int32(5);int32(32);int32(4);int32(3);int32(2);int32(1);int32(0);int32(15)]')  SignalSizes=str2num('[int32(1);int32(1);int32(1);int32(1);int32(1);int32(1);int32(1);int32(1);int32(1);int32(1);int32(1);int32(1);int32(1);int32(1);int32(1);int32(1);int32(1);int32(1);int32(1);int32(1);int32(1);int32(1);int32(1);int32(1);int32(1);int32(1);int32(1);int32(1);int32(1);int32(1);int32(1);int32(1);int32(1);int32(1);int32(1);int32(1);int32(1);int32(1);int32(1);int32(1)]')  ByteOrders=str2num('[int32(2);int32(2);int32(2);int32(2);int32(2);int32(2);int32(2);int32(2);int32(2);int32(2);int32(2);int32(2);int32(2);int32(2);int32(2);int32(2);int32(2);int32(2);int32(2);int32(2);int32(2);int32(2);int32(2);int32(2);int32(2);int32(2);int32(2);int32(2);int32(2);int32(2);int32(2);int32(2);int32(2);int32(2);int32(2);int32(2);int32(2);int32(2);int32(2);int32(2)]')  DataTypes=str2num('[int32(2);int32(2);int32(2);int32(2);int32(2);int32(2);int32(2);int32(2);int32(2);int32(2);int32(2);int32(2);int32(2);int32(2);int32(2);int32(2);int32(2);int32(2);int32(2);int32(2);int32(2);int32(2);int32(2);int32(2);int32(2);int32(2);int32(2);int32(2);int32(2);int32(2);int32(2);int32(2);int32(2);int32(2);int32(2);int32(2);int32(2);int32(2);int32(2);int32(2)]')  MultiplexTypes=str2num('[int32(1);int32(1);int32(1);int32(1);int32(1);int32(1);int32(1);int32(1);int32(1);int32(1);int32(1);int32(1);int32(1);int32(1);int32(1);int32(1);int32(1);int32(1);int32(1);int32(1);int32(1);int32(1);int32(1);int32(1);int32(1);int32(1);int32(1);int32(1);int32(1);int32(1);int32(1);int32(1);int32(1);int32(1);int32(1);int32(1);int32(1);int32(1);int32(1);int32(1)]')  MultiplexValues=str2num('[double(0);double(0);double(0);double(0);double(0);double(0);double(0);double(0);double(0);double(0);double(0);double(0);double(0);double(0);double(0);double(0);double(0);double(0);double(0);double(0);double(0);double(0);double(0);double(0);double(0);double(0);double(0);double(0);double(0);double(0);double(0);double(0);double(0);double(0);double(0);double(0);double(0);double(0);double(0);double(0)]')  Factors=str2num('[double(1);double(1);double(1);double(1);double(1);double(1);double(1);double(1);double(1);double(1);double(1);double(1);double(1);double(1);double(1);double(1);double(1);double(1);double(1);double(1);double(1);double(1);double(1);double(1);double(1);double(1);double(1);double(1);double(1);double(1);double(1);double(1);double(1);double(1);double(1);double(1);double(1);double(1);double(1);double(1)]')  Offsets=str2num('[double(0);double(0);double(0);double(0);double(0);double(0);double(0);double(0);double(0);double(0);double(0);double(0);double(0);double(0);double(0);double(0);double(0);double(0);double(0);double(0);double(0);double(0);double(0);double(0);double(0);double(0);double(0);double(0);double(0);double(0);double(0);double(0);double(0);double(0);double(0);double(0);double(0);double(0);double(0);double(0)]')  Minimums=str2num('[double(0);double(0);double(0);double(0);double(0);double(0);double(0);double(0);double(0);double(0);double(0);double(0);double(0);double(0);double(0);double(0);double(0);double(0);double(0);double(0);double(0);double(0);double(0);double(0);double(0);double(0);double(0);double(0);double(0);double(0);double(0);double(0);double(0);double(0);double(0);double(0);double(0);double(0);double(0);double(0)]')  Maximums=str2num('[double(1);double(1);double(1);double(1);double(1);double(1);double(1);double(1);double(1);double(1);double(1);double(1);double(1);double(1);double(1);double(1);double(1);double(1);double(1);double(1);double(1);double(1);double(1);double(1);double(1);double(1);double(1);double(1);double(1);double(1);double(1);double(1);double(1);double(1);double(1);double(1);double(1);double(1);double(1);double(1)]')
      settings: DataFormat=CANdb specified signals
  Mux : Mux  Inputs=8
  Mux1 : Mux  Inputs=6
  Mux2 : Mux  Inputs=10
  Mux3 : Mux  Inputs=10
  Mux4 : Mux  Inputs=10
  cb_cmds : Outport
  wires:
  CANB_Msg/1 -> [CANB_Msg]
  [CANB_Msg] -> CAN Unpack/1
  CAN Unpack/35 -> Mux1/1
  CAN Unpack/36 -> Mux1/2
  CAN Unpack/37 -> Mux1/3
  CAN Unpack/38 -> Mux1/4
  CAN Unpack/39 -> Mux1/5
  CAN Unpack/40 -> Mux1/6
  CAN Unpack/1 -> Mux2/1
  CAN Unpack/2 -> Mux2/2
  CAN Unpack/3 -> Mux2/3
  CAN Unpack/4 -> Mux2/4
  CAN Unpack/5 -> Mux2/5
  CAN Unpack/6 -> Mux2/6
  CAN Unpack/7 -> Mux2/7
  CAN Unpack/8 -> Mux2/8
  CAN Unpack/9 -> Mux2/9
  CAN Unpack/10 -> Mux2/10
  Mux1/1 -> [cell4_9]
  Mux2/1 -> [cell10_19]
  CAN Unpack/12 -> Mux3/1
  CAN Unpack/13 -> Mux3/2
  CAN Unpack/14 -> Mux3/3
  CAN Unpack/15 -> Mux3/4
  CAN Unpack/16 -> Mux3/5
  CAN Unpack/17 -> Mux3/6
  CAN Unpack/18 -> Mux3/7
  CAN Unpack/19 -> Mux3/8
  CAN Unpack/20 -> Mux3/9
  CAN Unpack/21 -> Mux3/10
  Mux3/1 -> [cell20_29]
  CAN Unpack/23 -> Mux4/1
  CAN Unpack/24 -> Mux4/2
  CAN Unpack/25 -> Mux4/3
  CAN Unpack/26 -> Mux4/4
  CAN Unpack/27 -> Mux4/5
  CAN Unpack/28 -> Mux4/6
  CAN Unpack/29 -> Mux4/7
  CAN Unpack/30 -> Mux4/8
  CAN Unpack/31 -> Mux4/9
  CAN Unpack/32 -> Mux4/10
  Mux4/1 -> [cell30_39]
  CAN Unpack/11 -> Mux/1
  CAN Unpack/22 -> Mux/2
  CAN Unpack/33 -> Mux/3
  [cell4_9] -> Mux/4
  [cell10_19] -> Mux/5
  [cell20_29] -> Mux/6
  [cell30_39] -> Mux/7
  CAN Unpack/34 -> Mux/8
  Mux/1 -> cb_cmds/1
